simulink model "sldemo_mdlref_bus"  (R2017b)
settings: Solver=FixedStepDiscrete  StartTime=0.0  StopTime=30  FixedStep=0.1  RelTol=1e-3  EnableMultiTasking=on
PreLoadFcn:
  | load sldemo_mdlref_counter_bus.mat
undefined symbols (not defined in the file or in its folder): sigbuilder_block
settings Model: ModifiedByFormat=The MathWorks Inc.  ExtModeAutoUpdateStatusClock=off  Creator=The MathWorks, Inc.  LastModifiedBy=The MathWorks Inc.
settings DataIOCC: SaveOutput=off  SaveTime=off  SignalLoggingName=topOut
settings OptimizationCC: DefaultParameterBehavior=Inlined  InlineInvariantSignals=on  ExpressionDepthLimit=2147483647  InitFltsAndDblsToZero=on  LifeSpan=inf
settings DebuggingCC: SaveWithParameterizedLinksMsg=none  UnderspecifiedInitializationDetection=Classic  MergeDetectMultiDrivingBlocksExec=none  CheckExecutionContextPreStartOutputMsg=on  CheckExecutionContextRuntimeOutputMsg=on  MultiTaskDSMMsg=warning  MultiTaskCondExecSysMsg=none  SigSpecEnsureSampleTimeMsg=none  FcnCallInpInsideContextMsg=warning  BusObjectLabelMismatch=error  AllowSymbolicDim=off  ModelReferenceDataLoggingMessage=none  StateNameClashWarn=warning  StrictBusMsg=ErrorOnBusTreatedAsVector  SFUnexpectedBacktrackingDiag=warning  SFNoUnconditionalDefaultTransitionDiag=warning  SFExecutionAtInitializationDiag=none
settings HardwareCC: ProdBitPerPointer=32  ProdBitPerSizeT=32  ProdBitPerPtrDiffT=32  ProdLargestAtomicFloat=None  ProdIntDivRoundTo=Undefined  ProdEndianess=Unspecified  ProdWordSize=32  ProdHWDeviceType=32-bit Generic  TargetHWDeviceType=32-bit Generic
settings ModelReferenceCC: UpdateModelReferenceTargets=IfOutOfDate  PropagateSignalLabelsOutOfModel=off
settings RTWCC: Description=Generic Real-Time Target  GenerateReport=on  LaunchReport=on
settings CodeAppCC: MaxIdLength=100  StateflowObjectComments=on
settings GRTTargetCC: TargetFcnLib=ansi_tfl_tmw.mat  TargetLangStandard=C89/C90 (ANSI)  GeneratePreprocessorConditionals=Disable all  CombineOutputUpdateFcns=off  MatFileLogging=off  GRTInterface=on
settings ConfigComp: CovMetricSettings=dw  CovHtmlReporting=on  CovSaveCumulativeToWorkspaceVar=on  CovSaveSingleToWorkspaceVar=on  CovExternalEMLEnable=off  CovSFcnEnable=off

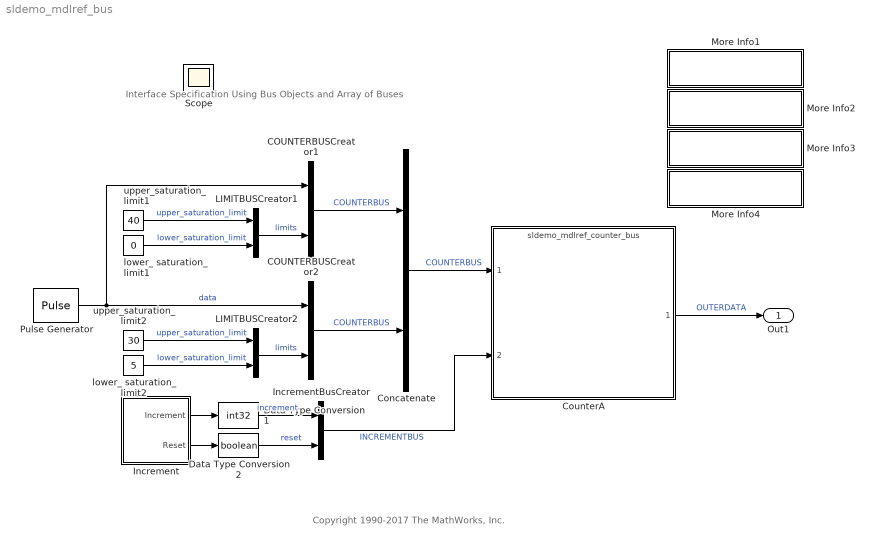
== system sldemo_mdlref_bus ==
  note: Interface Specification Using Bus Objects and Array of Buses
  note: Copyright 1990-2017 The MathWorks, Inc.
  COUNTERBUSCreator1 : BusCreator  Inputs=2  OutDataTypeStr=Bus: COUNTERBUS  NonVirtualBus=on
  COUNTERBUSCreator2 : BusCreator  Inputs=2  OutDataTypeStr=Bus: COUNTERBUS  NonVirtualBus=on
  Concatenate : Concatenate  Mode=Multidimensional array
  CounterA : ModelReference  ModelNameDialog=sldemo_mdlref_counter_bus  SimulationMode=Normal  ModelReferenceVersion=1.267
  Data Type Conversion1 : DataTypeConversion  OutDataTypeStr=int32
  Data Type Conversion2 : DataTypeConversion  OutDataTypeStr=boolean
  Increment : Subsystem  Tag=STV Subsys  LoadFcn=sigbuilder_block('load');  StartFcn=sigbuilder_block('start');  StopFcn=sigbuilder_block('stop');  ClipboardFcn=sigbuilder_block('clipboard');  mask(Sigbuilder block){tuvar=[0:10]}
      mask help: Create and generate interchangeable groups of signals whose waveforms are piecewise linear.
      mask init:
      | if ~strcmp(get_param(bdroot(gcbh),'SimulationStatus'),'stopped') tuvar = sigbuilder_block('maskInit'); end
      settings: CopyFcn=sigbuilder_block('copy');  DeleteFcn=sigbuilder_block('delete');  ModelCloseFcn=sigbuilder_block('modelClose');  PreSaveFcn=sigbuilder_block('preSave');  PauseFcn=sigbuilder_block('pause')  ContinueFcn=sigbuilder_block('continue')  NameChangeFcn=sigbuilder_block('namechange');  OpenFcn=sigbuilder_block('open',[3.2 253.6 1076.8 584 ]);  CloseFcn=sigbuilder_block('close');
      mask Display: plot(0, 0, 100, 100,[2, 2, 32, 32, 2], [68, 8, 8, 68, 68],[32, 2], [38, 38], [32, 19, 2],[53, 60, 44], [32, 17, 17, 2],[16, 16, 31, 31]);txt = getActiveGroup(gcbh);text(2, 100, txt,'verticalAlignment', 'top');
  IncrementBusCreator : BusCreator  Inputs=2  OutDataTypeStr=Bus: INCREMENTBUS  NonVirtualBus=on
  LIMITBUSCreator1 : BusCreator  Inputs=2  OutDataTypeStr=Bus: LIMITBUS  NonVirtualBus=on
  LIMITBUSCreator2 : BusCreator  Inputs=2  OutDataTypeStr=Bus: LIMITBUS  NonVirtualBus=on
  More Info1 : Subsystem
      settings: OpenFcn=helpview(fullfile(docroot,'simulink','helptargets.map'),'sldemo_mdlref_bus')
      mask Display: disp('Interface Specification')
  More Info2 : Subsystem
      settings: OpenFcn=helpview(fullfile(docroot,'simulink','helptargets.map'),'sldemo_mdlref_protect')
      mask Display: disp('Protected Models')
  More Info3 : Subsystem
      settings: OpenFcn=helpview(fullfile(docroot,'simulink','helptargets.map'),'sldemo_mdlref_logging_intervals')
      mask Display: disp('Logging Intervals')
  More Info4 : Subsystem
      settings: OpenFcn=helpview(fullfile(docroot,'simulink','helptargets.map'),'sldemo_working_with_big_data')
      mask Display: disp('Working with Big Data')
  Pulse Generator : DiscretePulseGenerator  Amplitude=int32(1)  SampleTime=0.1
  lower_ saturation_ limit1 : Constant  Value=0  OutDataTypeStr=int32
  lower_ saturation_ limit2 : Constant  Value=5  OutDataTypeStr=int32
  upper_saturation_limit1 : Constant  Value=40  OutDataTypeStr=int32
  upper_saturation_limit2 : Constant  Value=30  OutDataTypeStr=int32
  Out1 : Outport
  Scope : Scope
  wires:
  Concatenate/1 -> CounterA/1  "COUNTERBUS"
  CounterA/1 -> Out1/1  "OUTERDATA"
  Increment/1(Increment) -> Data Type Conversion1/1
  Data Type Conversion1/1 -> IncrementBusCreator/1  "increment"
  Data Type Conversion2/1 -> IncrementBusCreator/2  "reset"
  Increment/2(Reset) -> Data Type Conversion2/1
  IncrementBusCreator/1 -> CounterA/2  "INCREMENTBUS"
  COUNTERBUSCreator1/1 -> Concatenate/1  "COUNTERBUS"
  LIMITBUSCreator1/1 -> COUNTERBUSCreator1/2  "limits"
  COUNTERBUSCreator2/1 -> Concatenate/2  "COUNTERBUS"
  LIMITBUSCreator2/1 -> COUNTERBUSCreator2/2  "limits"
  upper_saturation_limit1/1 -> LIMITBUSCreator1/1  "upper_saturation_limit"
  lower_ saturation_ limit1/1 -> LIMITBUSCreator1/2  "lower_saturation_limit"
  Pulse Generator/1 -> COUNTERBUSCreator1/1, COUNTERBUSCreator2/1  "data"
  upper_saturation_limit2/1 -> LIMITBUSCreator2/1  "upper_saturation_limit"
  lower_ saturation_ limit2/1 -> LIMITBUSCreator2/2  "lower_saturation_limit"

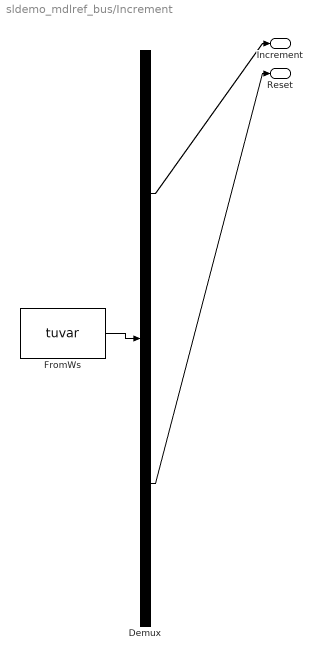
== system sldemo_mdlref_bus/Increment ==
  Demux : Demux  Tag=STV Demux  Outputs=2
  FromWs : FromWorkspace  Tag=STV FromWs  VariableName=tuvar  SampleTime=0.1  OutputAfterFinalValue=Holding final value
      SigBuilderData=|
      | common.afterFinalStr = 'Hold final value'
      | common.sampleTime = '0.1'
      | dataSet.timeRange = [0 30]
      | dataSet.name = 'Group 1'
      | sbobj.Groups.Name = 'Group 1'
      | sbobj.Groups.Signals(1).Name = 'Increment'
      | sbobj.Groups.Signals(1).XData = [0 15 15.1 30]
      | sbobj.Groups.Signals(1).YData = [1 1 -1 -1]
      | sbobj.Groups.Signals(2).Name = 'Reset'
      | sbobj.Groups.Signals(2).XData = [0 9.9 10 10.1 19.9 20 20.1 30]
      | sbobj.Groups.Signals(2).YData = [0 0 0.995 0 0 1 0 0]
      | sbobj.Groups.TimeRange = [0 30]
  Increment : Outport  Tag=STV Outport
  Reset : Outport  Tag=STV Outport  Port=2
  wires:
  FromWs/1 -> Demux/1
  Demux/1 -> Increment/1
  Demux/2 -> Reset/1

== system sldemo_mdlref_bus/More Info1 ==
  note: This demonstration shows how signals may be grouped and ungrouped while
      | retaining their names.  In this demonstration, 5 signals are created and labeled
      | appropriately.  These signals are then grouped together to create a bus of signals.
      | This bus of signals is then fed into the Bus Selector block.  Inside of the Bus
      | Selector block, the Pulse and Chirp signals are chosen to be output from the
      | original signal bus.
      |
      | It is possible to place a nest signal buses and then still retrieve the original signal
      | with its label.
  note: Bus Block Demonstration

== system sldemo_mdlref_bus/More Info2 ==
  note: Bus Block Demonstration
  note: This demonstration shows how signals may be grouped and ungrouped while
      | retaining their names.  In this demonstration, 5 signals are created and labeled
      | appropriately.  These signals are then grouped together to create a bus of signals.
      | This bus of signals is then fed into the Bus Selector block.  Inside of the Bus
      | Selector block, the Pulse and Chirp signals are chosen to be output from the
      | original signal bus.
      |
      | It is possible to place a nest signal buses and then still retrieve the original signal
      | with its label.

== system sldemo_mdlref_bus/More Info3 ==
  note: This demonstration shows how signals may be grouped and ungrouped while
      | retaining their names.  In this demonstration, 5 signals are created and labeled
      | appropriately.  These signals are then grouped together to create a bus of signals.
      | This bus of signals is then fed into the Bus Selector block.  Inside of the Bus
      | Selector block, the Pulse and Chirp signals are chosen to be output from the
      | original signal bus.
      |
      | It is possible to place a nest signal buses and then still retrieve the original signal
      | with its label.
  note: Bus Block Demonstration

== system sldemo_mdlref_bus/More Info4 ==
  note: Bus Block Demonstration
  note: This demonstration shows how signals may be grouped and ungrouped while
      | retaining their names.  In this demonstration, 5 signals are created and labeled
      | appropriately.  These signals are then grouped together to create a bus of signals.
      | This bus of signals is then fed into the Bus Selector block.  Inside of the Bus
      | Selector block, the Pulse and Chirp signals are chosen to be output from the
      | original signal bus.
      |
      | It is possible to place a nest signal buses and then still retrieve the original signal
      | with its label.
